simulink model "sm_aileron_actuator_2"  (R2022b)
settings: Solver=FixedStepAuto  StartTime=0.0  StopTime=50.0  FixedStep=0.01  RelTol=1e-3  AbsTol=1e-4  EnableMultiTasking=on
PostLoadFcn:
  | warning('off','sm:sli:setup:compile:LocalSolverNotSupported')
StartFcn:
  | tic
StopFcn:
  | Elapsed_Sim_Time = toc;
model workspace: external: MATLAB File aileronAssembly_DataFile.m (data not in the file)
undefined symbols (not defined in the file or in its folder): AAC_Param, ang2Ext_coeff, Ki, Ki_scaling_elec, Kp, Leadscrew, motor_friction, R7_sctrl, sigbuilder_block, sm_aileron_actuator_lib, smiData, X, Y, Z
libraries: sm_lib x608, fl_lib x380, ee_lib x103, nesl_utility x87, sh_lib x7, sdl_lib x3, simulink x2, slpidlib x2
(part 2 of 22)

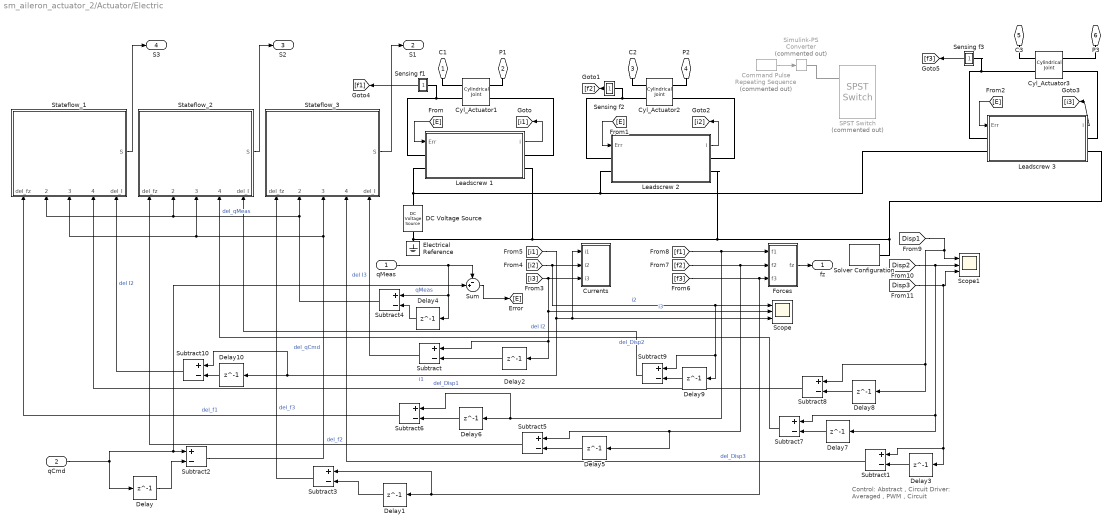
== system sm_aileron_actuator_2/Actuator/Electric ==
  note: Control: Abstract , Circuit
      | Driver: Averaged , PWM , Circuit
  qMeas : Inport
  "qCmd " : Inport  Port=2
  Command Pulse : simulink/Sources/Repeating Sequence  Commented=on  rep_seq_t="[0.0  4.0  6.0   8.0     10.0     12.0   14.0  16.0  18.0  20.0    22.0   24.0    26.0   28.0  30.0   32.0  34.0  36.0   38.0  40.0  42.0  44.0  46.0  48.0]"  rep_seq_y="[1.0  1.0  1.0  1.0  1.0  1.0  1.0  1.0  0.0  0.0  0.0  1.0  1.0  1.0  1.0   1.0  0.0  0.0  0.0  1.0  1.0  1.0  1.0  1.0]"
  Currents : Subsystem
  Cyl_Actuator1 : sm_lib/Joints/Cylindrical Joint  JointMode=Normal  SenseConstraintForce=off  SenseConstraintForceX=off  SenseConstraintForceY=off  SenseConstraintForceZ=off  SenseConstraintTorque=off  SenseConstraintTorqueX=off  SenseConstraintTorqueY=off  SenseConstraintTorqueZ=off  SenseTotalForce=off  SenseTotalForceX=off  SenseTotalForceY=off  SenseTotalForceZ=off  SenseTotalTorque=off  SenseTotalTorqueX=off  SenseTotalTorqueY=off  SenseTotalTorqueZ=off  CompositeWrenchDir=FollowerOnBase  CompositeWrenchFrame=BaseFrame  PzEquilibriumPosition=AAC_Param.Act.El.Spr.l0  PzEquilibriumPositionUnits=m  PzSpringStiffness=AAC_Param.Act.El.Spr.k  PzSpringStiffnessUnits=N/m  PzDampingCoefficient=AAC_Param.Act.El.Spr.b  PzDampingCoefficientUnits=N/(m/s)  PzTorqueActuationMode=InputTorque  PzMotionActuationMode=ComputedMotion  PzSensePosition=off  PzSenseVelocity=on  PzSenseAcceleration=off  PzSenseTorqueForce=off  PzSenseLowerLimitTorqueForce=off  PzSenseUpperLimitTorqueForce=off  PzLowerLimitSpecify=off  PzLowerLimitBound=-1  PzLowerLimitBoundUnits=m  PzLowerLimitStiffness=1e6  PzLowerLimitStiffnessUnits=N/m  PzLowerLimitDamping=1e3  PzLowerLimitDampingUnits=N/(m/s)  PzLowerLimitTransitionRegionWidth=1e-4  PzLowerLimitTransitionRegionWidthUnits=m  PzUpperLimitSpecify=off  PzUpperLimitBound=1  PzUpperLimitBoundUnits=m  PzUpperLimitStiffness=1e6  PzUpperLimitStiffnessUnits=N/m  PzUpperLimitDamping=1e3  PzUpperLimitDampingUnits=N/(m/s)  PzUpperLimitTransitionRegionWidth=1e-4  PzUpperLimitTransitionRegionWidthUnits=m  PzPositionTargetSpecify=on  PzPositionTargetPriority=Low  PzPositionTargetValue=smiData.CylindricalJoint(3).Pz.Pos  PzPositionTargetValueUnits=m  PzVelocityTargetSpecify=off  PzVelocityTargetPriority=High  PzVelocityTargetValue=0  PzVelocityTargetValueUnits=m/s  RzEquilibriumPosition=0  RzEquilibriumPositionUnits=rad  RzSpringStiffness=0  RzSpringStiffnessUnits=N*m/rad  RzDampingCoefficient=0  RzDampingCoefficientUnits=N*m/(rad/s)  RzTorqueActuationMode=NoTorque  RzMotionActuationMode=ComputedMotion  RzSensePosition=off  RzSenseVelocity=off  RzSenseAcceleration=off  RzSenseTorqueForce=off  RzSenseLowerLimitTorqueForce=off  RzSenseUpperLimitTorqueForce=off  RzLowerLimitSpecify=off  RzLowerLimitBound=-90  RzLowerLimitBoundUnits=deg  RzLowerLimitStiffness=1e4  RzLowerLimitStiffnessUnits=N*m/deg  RzLowerLimitDamping=10  RzLowerLimitDampingUnits=N*m/(deg/s)  RzLowerLimitTransitionRegionWidth=0.1  RzLowerLimitTransitionRegionWidthUnits=deg  RzUpperLimitSpecify=off  RzUpperLimitBound=90  RzUpperLimitBoundUnits=deg  RzUpperLimitStiffness=1e4  RzUpperLimitStiffnessUnits=N*m/deg  RzUpperLimitDamping=10  RzUpperLimitDampingUnits=N*m/(deg/s)  RzUpperLimitTransitionRegionWidth=0.1  RzUpperLimitTransitionRegionWidthUnits=deg  RzPositionTargetSpecify=on  RzPositionTargetPriority=Low  RzPositionTargetValue=smiData.CylindricalJoint(3).Rz.Pos  RzPositionTargetValueUnits=deg  RzVelocityTargetSpecify=off  RzVelocityTargetPriority=High  RzVelocityTargetValue=0  RzVelocityTargetValueUnits=deg/s
  Cyl_Actuator2 : sm_lib/Joints/Cylindrical Joint  JointMode=Normal  SenseConstraintForce=off  SenseConstraintForceX=off  SenseConstraintForceY=off  SenseConstraintForceZ=off  SenseConstraintTorque=off  SenseConstraintTorqueX=off  SenseConstraintTorqueY=off  SenseConstraintTorqueZ=off  SenseTotalForce=off  SenseTotalForceX=off  SenseTotalForceY=off  SenseTotalForceZ=off  SenseTotalTorque=off  SenseTotalTorqueX=off  SenseTotalTorqueY=off  SenseTotalTorqueZ=off  CompositeWrenchDir=FollowerOnBase  CompositeWrenchFrame=BaseFrame  PzEquilibriumPosition=AAC_Param.Act.El.Spr.l0  PzEquilibriumPositionUnits=m  PzSpringStiffness=AAC_Param.Act.El.Spr.k  PzSpringStiffnessUnits=N/m  PzDampingCoefficient=AAC_Param.Act.El.Spr.b  PzDampingCoefficientUnits=N/(m/s)  PzTorqueActuationMode=InputTorque  PzMotionActuationMode=ComputedMotion  PzSensePosition=off  PzSenseVelocity=on  PzSenseAcceleration=off  PzSenseTorqueForce=off  PzSenseLowerLimitTorqueForce=off  PzSenseUpperLimitTorqueForce=off  PzLowerLimitSpecify=off  PzLowerLimitBound=-1  PzLowerLimitBoundUnits=m  PzLowerLimitStiffness=1e6  PzLowerLimitStiffnessUnits=N/m  PzLowerLimitDamping=1e3  PzLowerLimitDampingUnits=N/(m/s)  PzLowerLimitTransitionRegionWidth=1e-4  PzLowerLimitTransitionRegionWidthUnits=m  PzUpperLimitSpecify=off  PzUpperLimitBound=1  PzUpperLimitBoundUnits=m  PzUpperLimitStiffness=1e6  PzUpperLimitStiffnessUnits=N/m  PzUpperLimitDamping=1e3  PzUpperLimitDampingUnits=N/(m/s)  PzUpperLimitTransitionRegionWidth=1e-4  PzUpperLimitTransitionRegionWidthUnits=m  PzPositionTargetSpecify=on  PzPositionTargetPriority=Low  PzPositionTargetValue=smiData.CylindricalJoint(2).Pz.Pos  PzPositionTargetValueUnits=m  PzVelocityTargetSpecify=off  PzVelocityTargetPriority=High  PzVelocityTargetValue=0  PzVelocityTargetValueUnits=m/s  RzEquilibriumPosition=0  RzEquilibriumPositionUnits=rad  RzSpringStiffness=0  RzSpringStiffnessUnits=N*m/rad  RzDampingCoefficient=0  RzDampingCoefficientUnits=N*m/(rad/s)  RzTorqueActuationMode=NoTorque  RzMotionActuationMode=ComputedMotion  RzSensePosition=off  RzSenseVelocity=off  RzSenseAcceleration=off  RzSenseTorqueForce=off  RzSenseLowerLimitTorqueForce=off  RzSenseUpperLimitTorqueForce=off  RzLowerLimitSpecify=off  RzLowerLimitBound=-90  RzLowerLimitBoundUnits=deg  RzLowerLimitStiffness=1e4  RzLowerLimitStiffnessUnits=N*m/deg  RzLowerLimitDamping=10  RzLowerLimitDampingUnits=N*m/(deg/s)  RzLowerLimitTransitionRegionWidth=0.1  RzLowerLimitTransitionRegionWidthUnits=deg  RzUpperLimitSpecify=off  RzUpperLimitBound=90  RzUpperLimitBoundUnits=deg  RzUpperLimitStiffness=1e4  RzUpperLimitStiffnessUnits=N*m/deg  RzUpperLimitDamping=10  RzUpperLimitDampingUnits=N*m/(deg/s)  RzUpperLimitTransitionRegionWidth=0.1  RzUpperLimitTransitionRegionWidthUnits=deg  RzPositionTargetSpecify=on  RzPositionTargetPriority=Low  RzPositionTargetValue=smiData.CylindricalJoint(2).Rz.Pos  RzPositionTargetValueUnits=deg  RzVelocityTargetSpecify=off  RzVelocityTargetPriority=High  RzVelocityTargetValue=0  RzVelocityTargetValueUnits=deg/s
  Cyl_Actuator3 : sm_lib/Joints/Cylindrical Joint  JointMode=Normal  SenseConstraintForce=off  SenseConstraintForceX=off  SenseConstraintForceY=off  SenseConstraintForceZ=off  SenseConstraintTorque=off  SenseConstraintTorqueX=off  SenseConstraintTorqueY=off  SenseConstraintTorqueZ=off  SenseTotalForce=off  SenseTotalForceX=off  SenseTotalForceY=off  SenseTotalForceZ=off  SenseTotalTorque=off  SenseTotalTorqueX=off  SenseTotalTorqueY=off  SenseTotalTorqueZ=off  CompositeWrenchDir=FollowerOnBase  CompositeWrenchFrame=BaseFrame  PzEquilibriumPosition=AAC_Param.Act.El.Spr.l0  PzEquilibriumPositionUnits=m  PzSpringStiffness=AAC_Param.Act.El.Spr.k  PzSpringStiffnessUnits=N/m  PzDampingCoefficient=AAC_Param.Act.El.Spr.b  PzDampingCoefficientUnits=N/(m/s)  PzTorqueActuationMode=InputTorque  PzMotionActuationMode=ComputedMotion  PzSensePosition=off  PzSenseVelocity=on  PzSenseAcceleration=off  PzSenseTorqueForce=off  PzSenseLowerLimitTorqueForce=off  PzSenseUpperLimitTorqueForce=off  PzLowerLimitSpecify=off  PzLowerLimitBound=-1  PzLowerLimitBoundUnits=m  PzLowerLimitStiffness=1e6  PzLowerLimitStiffnessUnits=N/m  PzLowerLimitDamping=1e3  PzLowerLimitDampingUnits=N/(m/s)  PzLowerLimitTransitionRegionWidth=1e-4  PzLowerLimitTransitionRegionWidthUnits=m  PzUpperLimitSpecify=off  PzUpperLimitBound=1  PzUpperLimitBoundUnits=m  PzUpperLimitStiffness=1e6  PzUpperLimitStiffnessUnits=N/m  PzUpperLimitDamping=1e3  PzUpperLimitDampingUnits=N/(m/s)  PzUpperLimitTransitionRegionWidth=1e-4  PzUpperLimitTransitionRegionWidthUnits=m  PzPositionTargetSpecify=on  PzPositionTargetPriority=Low  PzPositionTargetValue=smiData.CylindricalJoint(1).Pz.Pos  PzPositionTargetValueUnits=m  PzVelocityTargetSpecify=off  PzVelocityTargetPriority=High  PzVelocityTargetValue=0  PzVelocityTargetValueUnits=m/s  RzEquilibriumPosition=0  RzEquilibriumPositionUnits=rad  RzSpringStiffness=0  RzSpringStiffnessUnits=N*m/rad  RzDampingCoefficient=0  RzDampingCoefficientUnits=N*m/(rad/s)  RzTorqueActuationMode=NoTorque  RzMotionActuationMode=ComputedMotion  RzSensePosition=off  RzSenseVelocity=off  RzSenseAcceleration=off  RzSenseTorqueForce=off  RzSenseLowerLimitTorqueForce=off  RzSenseUpperLimitTorqueForce=off  RzLowerLimitSpecify=off  RzLowerLimitBound=-90  RzLowerLimitBoundUnits=deg  RzLowerLimitStiffness=1e4  RzLowerLimitStiffnessUnits=N*m/deg  RzLowerLimitDamping=10  RzLowerLimitDampingUnits=N*m/(deg/s)  RzLowerLimitTransitionRegionWidth=0.1  RzLowerLimitTransitionRegionWidthUnits=deg  RzUpperLimitSpecify=off  RzUpperLimitBound=90  RzUpperLimitBoundUnits=deg  RzUpperLimitStiffness=1e4  RzUpperLimitStiffnessUnits=N*m/deg  RzUpperLimitDamping=10  RzUpperLimitDampingUnits=N*m/(deg/s)  RzUpperLimitTransitionRegionWidth=0.1  RzUpperLimitTransitionRegionWidthUnits=deg  RzPositionTargetSpecify=on  RzPositionTargetPriority=Low  RzPositionTargetValue=smiData.CylindricalJoint(1).Rz.Pos  RzPositionTargetValueUnits=deg  RzVelocityTargetSpecify=off  RzVelocityTargetPriority=High  RzVelocityTargetValue=0  RzVelocityTargetValueUnits=deg/s
  DC Voltage Source : fl_lib/Electrical/Electrical Sources/DC Voltage Source  v0=24 V
  Delay{,1..10} (11 alike) : Delay  DelayLength=1
  Electrical Reference : fl_lib/Electrical/Electrical Elements/Electrical Reference
  Forces : Subsystem
  Leadscrew 1 : Subsystem  AncestorBlock=sm_aileron_actuator_lib/Leadscrew  mask{popup_ctrl=Simulink, popup_driver=Averaged}
      mask prompts: popup_ctrl "Controller"; popup_driver "Driver Circuit"
      mask init:
      | if(popup_ctrl == 1)
      |     set_param([gcb '/Control'],'OverrideUsingVariant','Simulink')
      | else
      |     set_param([gcb '/Control'],'OverrideUsingVariant','Circuit')
      | end
      | 
      | if(popup_driver == 3)
      |     set_param([gcb '/Motor Driver'],'OverrideUsingVariant','Circuit')
      | else
      |     set_param([gcb '/Motor Driver'],'OverrideUsingVariant','Abstract')
      |     if(popup_driver == 1)
      |         set_param([gcb '/Motor Driver/Abstract/Controlled PWM Voltage'],'pwm_or_av','2');
      |         set_param([gcb '/Motor Driver/Abstract/H-Bridge'],'pwm_or_av','2');
      |     else
      |         set_param([gcb '/Motor Driver/Abstract/Controlled PWM Voltage'],'pwm_or_av','1');
      |         set_param([gcb '/Motor Driver/Abstract/H-Bridge'],'pwm_or_av','1');
      |     end
      | end
      | 
      | set_param([gcb '/Control'],'Name','Control');
      | set_param([gcb '/Motor Driver'],'Name','Motor Driver');
      settings: LibrarySourceBlock=sm_aileron_actuator_lib/Leadscrew
      mask TypeOptions popup_ctrl: Simulink | Circuit
      mask TypeOptions popup_driver: Averaged | PWM | Circuit
      mask Display:
      | SnC_Char = get_param(gcb,'popup_ctrl');
      | PWM_Char = get_param(gcb,'popup_driver');
      | 
      | try
      |     image(['sm_aileron_actuator_msc' upper(SnC_Char(1)) 'pw' PWM_Char(1) '_IMAGE.png']);
      | catch
      | 
      | end
  Leadscrew 2 : Subsystem  AncestorBlock=sm_aileron_actuator_lib/Leadscrew  mask{popup_ctrl=Simulink, popup_driver=Averaged}
      mask prompts: popup_ctrl "Controller"; popup_driver "Driver Circuit"
      mask init: same as sm_aileron_actuator_2/Actuator/Electric/Leadscrew 1
      settings: LibrarySourceBlock=sm_aileron_actuator_lib/Leadscrew
      mask TypeOptions popup_ctrl: Simulink | Circuit
      mask TypeOptions popup_driver: Averaged | PWM | Circuit
      mask Display:
      | SnC_Char = get_param(gcb,'popup_ctrl');
      | PWM_Char = get_param(gcb,'popup_driver');
      | 
      | try
      |     image(['sm_aileron_actuator_msc' upper(SnC_Char(1)) 'pw' PWM_Char(1) '_IMAGE.png']);
      | catch
      | 
      | end
  Leadscrew 3 : Subsystem  AncestorBlock=sm_aileron_actuator_lib/Leadscrew  mask{popup_ctrl=Simulink, popup_driver=Averaged}
      mask prompts: popup_ctrl "Controller"; popup_driver "Driver Circuit"
      mask init: same as sm_aileron_actuator_2/Actuator/Electric/Leadscrew 1
      settings: LibrarySourceBlock=sm_aileron_actuator_lib/Leadscrew
      mask TypeOptions popup_ctrl: Simulink | Circuit
      mask TypeOptions popup_driver: Averaged | PWM | Circuit
      mask Display:
      | SnC_Char = get_param(gcb,'popup_ctrl');
      | PWM_Char = get_param(gcb,'popup_driver');
      | 
      | try
      |     image(['sm_aileron_actuator_msc' upper(SnC_Char(1)) 'pw' PWM_Char(1) '_IMAGE.png']);
      | catch
      | 
      | end
  SPST Switch : ee_lib/Switches & Breakers/SPST Switch  Commented=on  R_closed=0.01 Ohm  G_open=1e-6 S  Threshold=0.5 V  Width=0 V  model_dynamics=0  t_on=1e-3 s  t_off=1e-3 s  initial_vT=0 V
      settings: InternalSimscapePortConfiguration="{\"Bottom\":[],\"Left\":[{\"id\":\"vT\",\"label\":\"vT\",\"type\":\"input\"},{\"id\":\"p\",\"label\":\"\",\"type\":\"foundation.electrical.electrical\"}],\"Right\":[{\"id\":\"n\",\"label\":\"\",\"type\":\"foundation.electrical.electrical\"}],\"Top\":[]}"
  Scope : Scope  NumInputPorts=3
  Scope1 : Scope  NumInputPorts=3
  Sensing f1 : Subsystem
      mask Display: disp(' ');
  Sensing f2 : Subsystem
      mask Display: disp(' ');
  Sensing f3 : Subsystem
      mask Display: disp(' ');
  Simulink-PS Converter : nesl_utility/Simulink-PS Converter  Commented=on  PhysicalDomain=network_engine_domain  SubClassName=ps_input  LeftPortType=input  RightPortType=output  PseudoPeriodic=off  Frequencies=[]  NoiseDistribution=none  NoiseParameters=[]  Unit=1  AffineConversion=off  FilteringAndDerivatives=provide  SimscapeFilterOrder=1  InputFilterTimeConstant=0.001  UdotUserProvided=0
  Solver Configuration : nesl_utility/Solver Configuration  PhysicalDomain=network_engine_domain  SubClassName=solver  LeftPortType=input  RightPortType=generic  Tones=[]  Harmonics=[]  SimulateNoise=off  Profile=off  UseLocalSampling=off  EnableSwitchedLinearOptims=on  FrequencyDomain=off  UseCCode=off  RelTol=0.001  AbsTol=1e-06  MinStep=1e-09  ToWorkspace=off  RevertToSquareIcSolve=off  NumHomotopyIterations=100  PhasorMode=off  PhasorModeNumHarmonics=1  ConsistencySolver=NEWTON_FTOL  IndexReductionMethod=DerivativeReplacement  DoDC=off  ResidualTolerance=1e-09  ConsistencyTolSource=GLOBAL  ConsistencyAbsTol=0.001  ConsistencyRelTol=0.001  ConsistencyTolFactor=0.001  UseLocalSolver=off  LocalSolverChoice=NE_BACKWARD_EULER_ADVANCER  ResolveIndetEquations=on  FunctionEvalNumThread=1  LocalSolverSampleTime=0.001  DoFixedCost=off  MaxNonlinIter=3  MaxModeIter=2  ComputeImpulses=off  ImpulseIterations=2  LinearAlgebra=Sparse  LinearAlgebraNumThread=0  EquationFormulation=NE_TIME_EF  DelaysMemoryBudget=1024  AutomaticFiltering=on  FilteringTimeConstant=0.001  PartitionStorageMethod=AS_NEEDED  PartitionMemoryBudget=1024  PartitionMethod=FAST
  Stateflow_1 : Stateflow chart  TreatAsAtomicUnit=on
      settings: PortSchema="{\"entries\":[{\"content\":{\"sides\":[{\"content\":{\"connectorIds\":[]},\"type\":\"ConnectorPlacement.EquallySpacedRectSide\",\"uuid\":\"e042e97c-c059-43b9-8a3a-af78b6eb416a\"},{\"content\":{\"connectorIds\":[\"Out1\"],\"side\":\"RIGHT\"},\"type\":\"ConnectorPlacement.EquallySpacedRectSide\",\"uuid\":\"2ca5b953-ef1b-4dff-bad4-a239d4259fe4\"},{\"content\":{\"connectorIds\":[],\"side\":\"TOP\"},\"type\":\"ConnectorPlacement.EquallySpacedRectSide\",\"uuid\":\"97c6fc3f-7b5c-403e-9b9f-ca095dc81ec0\"},{\"content\":{\"connectorIds\":[\"In1\",\"In2\",\"In3\",\"In4\",\"In5\"],\"side\":\"BOTTOM\"},\"type\":\"ConnectorPlacement.EquallySpacedRectSide\",\"uuid\":\"8bf8b472-13ff-4770-ba34-49bd9ed987ee\"}]},\"type\":\"ConnectorPlacement.EquallySpacedConnector\",\"uuid\":\"0dfcd544-5d90-4c16-a349-47b1199a081b\"}],\"packageUris\":[\"http://schema.mathworks.com/mf0/Connector/R2020b\"],\"version\":\"1.0\"}"
  Stateflow_2 : Stateflow chart  TreatAsAtomicUnit=on
      settings: PortSchema="{\"entries\":[{\"content\":{\"sides\":[{\"content\":{\"connectorIds\":[]},\"type\":\"ConnectorPlacement.EquallySpacedRectSide\",\"uuid\":\"e042e97c-c059-43b9-8a3a-af78b6eb416a\"},{\"content\":{\"connectorIds\":[\"Out1\"],\"side\":\"RIGHT\"},\"type\":\"ConnectorPlacement.EquallySpacedRectSide\",\"uuid\":\"2ca5b953-ef1b-4dff-bad4-a239d4259fe4\"},{\"content\":{\"connectorIds\":[],\"side\":\"TOP\"},\"type\":\"ConnectorPlacement.EquallySpacedRectSide\",\"uuid\":\"97c6fc3f-7b5c-403e-9b9f-ca095dc81ec0\"},{\"content\":{\"connectorIds\":[\"In1\",\"In2\",\"In3\",\"In4\",\"In5\"],\"side\":\"BOTTOM\"},\"type\":\"ConnectorPlacement.EquallySpacedRectSide\",\"uuid\":\"8bf8b472-13ff-4770-ba34-49bd9ed987ee\"}]},\"type\":\"ConnectorPlacement.EquallySpacedConnector\",\"uuid\":\"0dfcd544-5d90-4c16-a349-47b1199a081b\"}],\"packageUris\":[\"http://schema.mathworks.com/mf0/Connector/R2020b\"],\"version\":\"1.0\"}"
  Stateflow_3 : Stateflow chart  TreatAsAtomicUnit=on
      settings: PortSchema="{\"entries\":[{\"content\":{\"sides\":[{\"content\":{\"connectorIds\":[]},\"type\":\"ConnectorPlacement.EquallySpacedRectSide\",\"uuid\":\"e042e97c-c059-43b9-8a3a-af78b6eb416a\"},{\"content\":{\"connectorIds\":[\"Out1\"],\"side\":\"RIGHT\"},\"type\":\"ConnectorPlacement.EquallySpacedRectSide\",\"uuid\":\"2ca5b953-ef1b-4dff-bad4-a239d4259fe4\"},{\"content\":{\"connectorIds\":[],\"side\":\"TOP\"},\"type\":\"ConnectorPlacement.EquallySpacedRectSide\",\"uuid\":\"97c6fc3f-7b5c-403e-9b9f-ca095dc81ec0\"},{\"content\":{\"connectorIds\":[\"In1\",\"In2\",\"In3\",\"In4\",\"In5\"],\"side\":\"BOTTOM\"},\"type\":\"ConnectorPlacement.EquallySpacedRectSide\",\"uuid\":\"8bf8b472-13ff-4770-ba34-49bd9ed987ee\"}]},\"type\":\"ConnectorPlacement.EquallySpacedConnector\",\"uuid\":\"0dfcd544-5d90-4c16-a349-47b1199a081b\"}],\"packageUris\":[\"http://schema.mathworks.com/mf0/Connector/R2020b\"],\"version\":\"1.0\"}"
  Subtract{,1..10} (11 alike) : Sum  Inputs=+-
  Sum : Sum  Inputs=-+|
  C1 : PMIOPort  Side=Right
  P1 : PMIOPort  Port=2  Side=Right
  C2 : PMIOPort  Port=3  Side=Right
  P2 : PMIOPort  Port=4  Side=Right
  C3 : PMIOPort  Port=5  Side=Right
  P3 : PMIOPort  Port=6  Side=Right
  fz : Outport  VectorParamsAs1DForOutWhenUnconnected=off
  S1 : Outport  Port=2
  S2 : Outport  Port=3
  S3 : Outport  Port=4
  wires:
  Sum/1 -> [E]
  "qCmd "/1 -> Sum/2, Subtract2/1, Delay/1
  [E] -> Leadscrew 1/1(Err)
  [E] -> Leadscrew 2/1(Err)
  [E] -> Leadscrew 3/1(Err)
  Leadscrew 1/1(i) -> [i1]
  Leadscrew 2/1(i) -> [i2]
  Leadscrew 3/1(i) -> [i3]
  [i1] -> Subtract10/1, Delay10/1, Scope/3, Currents/1(i1)  "i1"
  [i2] -> Delay9/1, Subtract9/1, Scope/1, Currents/2(i2)  "i2"
  [i3] -> Delay2/1, Subtract/1, Scope/2, Currents/3(i3)  "i3"
  [f3] -> Subtract3/1, Delay1/1, Forces/3(f3)
  [f2] -> Delay5/1, Subtract5/1, Forces/2(f2)
  [f1] -> Subtract6/1, Delay6/1, Forces/1(f1)
  Forces/1(fz) -> fz/1
  Sensing f2/1(o) -> [f2]
  Sensing f1/1(o) -> [f1]
  Sensing f3/1(o) -> [f3]
  [Disp2] -> Subtract7/1, Delay7/1, Scope1/2
  [Disp1] -> Subtract8/1, Delay8/1, Scope1/1
  [Disp3] -> Delay3/1, Subtract1/1, Scope1/3
  Delay2/1 -> Subtract/2
  Subtract/1 -> Stateflow_3/5(del_I)  "del I3"
  Delay3/1 -> Subtract1/2
  Subtract1/1 -> Stateflow_3/4(del_Disp)  "del_Disp3"
  qMeas/1 -> Delay4/1, Subtract4/1, Sum/1  "qMeas"
  Subtract3/1 -> Stateflow_3/1(del_fz)  "del_f3"
  Delay1/1 -> Subtract3/2
  Stateflow_3/1(S) -> S1/1
  Delay/1 -> Subtract2/2
  Subtract2/1 -> Stateflow_1/3(del_qCmd), Stateflow_2/3(del_qCmd), Stateflow_3/3(del_qCmd)  "del_qCmd"
  Delay4/1 -> Subtract4/2
  Subtract4/1 -> Stateflow_1/2(del_qMeas), Stateflow_2/2(del_qMeas), Stateflow_3/2(del_qMeas)  "del_qMeas"
  Delay5/1 -> Subtract5/2
  Subtract5/1 -> Stateflow_2/1(del_fz)  "del_f2"
  Delay6/1 -> Subtract6/2
  Subtract6/1 -> Stateflow_1/1(del_fz)  "del_f1"
  Delay7/1 -> Subtract7/2
  Subtract7/1 -> Stateflow_2/4(del_Disp)  "del_Disp2"
  Delay8/1 -> Subtract8/2
  Subtract8/1 -> Stateflow_1/4(del_Disp)  "del_Disp1"
  Delay9/1 -> Subtract9/2
  Subtract9/1 -> Stateflow_2/5(del_I)  "del I2"
  Delay10/1 -> Subtract10/2
  Subtract10/1 -> Stateflow_1/5(del_I)  "del I2"
  Stateflow_2/1(S) -> S2/1
  Stateflow_1/1(S) -> S3/1
  Command Pulse/1 -> Simulink-PS Converter/1
  connections:
  Leadscrew 3/LConn1 -- Sensing f3/LConn1 -- Cyl_Actuator3/LConn2
  Leadscrew 3/RConn1 -- Cyl_Actuator3/RConn2
  Leadscrew 2/LConn1 -- Sensing f2/LConn1 -- Cyl_Actuator2/LConn2
  Leadscrew 1/LConn1 -- Sensing f1/LConn1 -- Cyl_Actuator1/LConn2
  Leadscrew 1/RConn1 -- Cyl_Actuator1/RConn2
  Cyl_Actuator3/LConn1 -- C3/RConn1
  Cyl_Actuator1/LConn1 -- C1/RConn1
  Cyl_Actuator3/RConn1 -- P3/RConn1
  Cyl_Actuator2/RConn1 -- P2/RConn1
  Cyl_Actuator1/RConn1 -- P1/RConn1
  Cyl_Actuator2/LConn1 -- C2/RConn1
  DC Voltage Source/LConn1 -- Leadscrew 1/LConn2 -- Leadscrew 3/LConn2 -- Leadscrew 2/LConn2
  Electrical Reference/LConn1 -- Leadscrew 3/RConn2 -- Solver Configuration/RConn1 -- Leadscrew 2/RConn2 -- Leadscrew 1/RConn2 -- DC Voltage Source/RConn1
  Cyl_Actuator2/RConn2 -- Leadscrew 2/RConn1
  Simulink-PS Converter/RConn1 -- SPST Switch/LConn1
